simulink model "rc_circuit"  (R2024b)
settings: Solver=FixedStepAuto  StartTime=0.0  StopTime=10.0  FixedStep=0.001  RelTol=1e-3
settings Model: Creator=Admin  LastModifiedBy=Admin

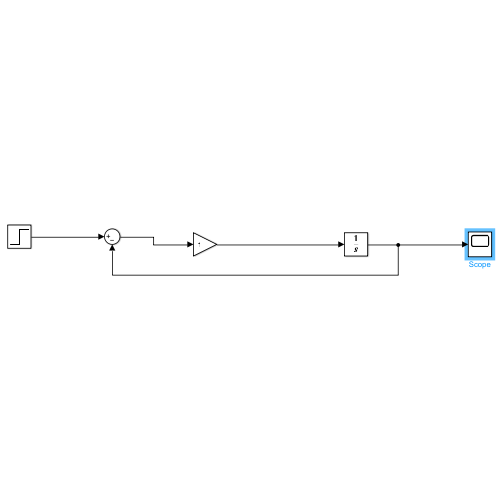
[thumbnail: Simulink's stored preview of the top-level diagram]
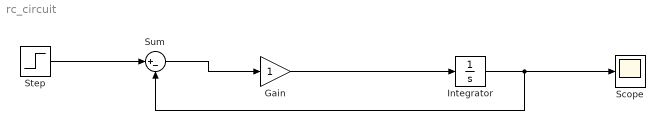
== system rc_circuit ==
  Gain : Gain
  Integrator : Integrator
  Scope : Scope
  Step : Step  Time=0  After=5  SampleTime=0
  Sum : Sum  Inputs=|+-
  wires:
  Integrator/1 -> Sum/2, Scope/1
  Step/1 -> Sum/1
  Gain/1 -> Integrator/1
  Sum/1 -> Gain/1
